simulink model "ScriptDemo"  (R2022b)
settings: configuration reference "TmVcThermal_Configuration_sub" (kept outside this file)
undefined symbols (not defined in the file): aaaa, bbbb, cTmComprCtrl_D_u8HvacFlowTable_db, cTmComprCtrl_D_u8HvacFlowTable_sw, cTmComprCtrl_n_i16ChillCmpIMax, cTmComprCtrl_n_i16ChillCmpIMin, cTmComprCtrl_n_i16ChillCmpIMin666, cTmComprCtrl_n_i16ChillCmpPMax, cTmComprCtrl_n_i16ChillCmpPMin, cTmComprCtrl_n_i16CmpChillCoolRpmKiMax, cTmComprCtrl_n_i16CmpChillCoolRpmKiMin, cTmComprCtrl_n_i16CmpChillCoolRpmKpMax, cTmComprCtrl_n_i16CmpChillCoolRpmKpMin, cTmComprCtrl_n_i16CmpCoolRpmKiMax, cTmComprCtrl_n_i16CmpCoolRpmKiMin, cTmComprCtrl_n_i16CmpCoolRpmKpMax, cTmComprCtrl_n_i16CmpCoolRpmKpMin, cTmComprCtrl_n_i16SM4CmpHeatKiMax, cTmComprCtrl_n_i16SM4CmpHeatKiMin, cTmComprCtrl_n_i16SM4CmpHeatKpMax, cTmComprCtrl_n_i16SM4CmpHeatKpMin, cTmComprCtrl_n_i16SM5CmpHeatKiMax, cTmComprCtrl_n_i16SM5CmpHeatKiMin, cTmComprCtrl_n_i16SM5CmpHeatKpMax, cTmComprCtrl_n_i16SM5CmpHeatKpMin, cTmComprCtrl_n_i16SM6CmpHeatKiMax, cTmComprCtrl_n_i16SM6CmpHeatKiMin, cTmComprCtrl_n_i16SM6CmpHeatKpMax, cTmComprCtrl_n_i16SM6CmpHeatKpMin, cTmComprCtrl_n_u16CmpMaxSpdFanFltLimt, cTmComprCtrl_n_u16CmpMaxSpdLoSidePFltLimt, cTmComprCtrl_n_u16CmpMaxSpdSensorFltLimt, cTmComprCtrl_n_u16CompMinRpm, cTmComprCtrl_n_u16CompRpmIncThres, cTmComprCtrl_t_u16BattCooltFFPeriod, cTmComprCtrl_t_u16BattCooltPIPeriod, cTmComprCtrl_t_u16CmpCoolFFPeriod, cTmComprCtrl_t_u16CmpCoolPIPeriod, cTmComprCtrl_t_u16CoolCmpChillFFPeriod, cTmComprCtrl_t_u16CoolCmpChillPIPeriod, cTmComprCtrl_t_u16SM4CmpHeatFFPeriod, cTmComprCtrl_t_u16SM4CmpHeatPIPeriod, cTmComprCtrl_t_u16SM5CmpHeatFFPeriod, cTmComprCtrl_t_u16SM5CmpHeatPIPeriod, cTmComprCtrl_t_u16SM6CmpHeatFFPeriod, cTmComprCtrl_t_u16SM6CmpHeatPIPeriod, cTmComprCtrl_Te_EvapClearInteg, cTmComprCtrl_Te_i16HpReqTempSaturoffset, cTmComprCtrl_Te_i16SatLpReplaceDiff, cTmComprCtrl_Te_i16SM3BatDiffStartEvapDecOffset, cTmComprCtrl_Te_i16SM3EvapLo, cTmComprCtrl_Te_i16SM3TBatDiffEntEvapDecOffset, cTmComprCtrl_Te_i16SM3TBatDiffEntEvapDecOffsetQuit, cTmComprCtrl_Te_s32ErrCmpChillPIContinueCoolH, cTmComprCtrl_Te_s32ErrCmpChillPIContinueCoolL, cTmComprCtrl_Te_s32ErrCmpPIContinueChillH, cTmComprCtrl_Te_s32ErrCmpPIContinueChillL, cTmComprCtrl_Te_s32ErrCmpPIContinueCoolH, cTmComprCtrl_Te_s32ErrCmpPIContinueCoolL, cTmComprCtrl_Te_s32ErrCmpPIContinueHeatH ... (+398)
libraries: simulink x782, PCMULib x640, simulink_need_slupdate x4
(part 20 of 41)

== system ScriptDemo/Create/createMerge/After/SM1SM21/ID26245_SM1FF ==
  sTmIn_Te_s32HvBattCooltTReq : Inport
  sTmIn_D_u8DCChrgSt : Inport  Port=2  OutDataTypeStr=uint8
  sTmSigProces_D_u8HvBattCoolgReq : Inport  Port=3  OutDataTypeStr=uint8
  sTmSigProces_Te_s32TAmb : Inport  Port=4  OutDataTypeStr=single
  sTmIn_D_u8HeatPump : Inport  Port=5  OutDataTypeStr=uint8
  Enable : EnablePort
  1-D Lookup Table : Lookup_n-D  NumberOfTableDimensions=1  BreakpointsForDimension1=tTmComprCtrl_fac_s32SM1FFTFactor_X  BreakpointsForDimension1DataTypeStr=Inherit: Inherit from 'Breakpoint data'  Table=tTmComprCtrl_fac_s32SM1FFTFactor  TableDataTypeStr=Inherit: Inherit from 'Table data'  ExtrapMethod=Clip  InternalRulePriority=Speed  OutDataTypeStr=Inherit: Inherit via back propagation  RndMeth=Simplest  InputSameDT=off
  2-D Lookup Table : Lookup_n-D  BreakpointsForDimension1=mTmComprCtrl_n_u16FFBattCooltRpmNorm_Y  BreakpointsForDimension2=mTmComprCtrl_n_u16FFBattCooltRpmNorm_X  BreakpointsForDimension1DataTypeStr=Inherit: Inherit from 'Breakpoint data'  BreakpointsForDimension2DataTypeStr=Inherit: Inherit from 'Breakpoint data'  Table=mTmComprCtrl_n_u16FFBattCooltRpmNorm  TableDataTypeStr=Inherit: Inherit from 'Table data'  ExtrapMethod=Clip  InternalRulePriority=Speed  OutDataTypeStr=Inherit: Inherit via back propagation  RndMeth=Simplest  InputSameDT=off
      settings: InputPortMap=u0,u1
  2-D Lookup Table1 : Lookup_n-D  BreakpointsForDimension1=mTmComprCtrl_n_u16FFBattCooltRpmNormNhp_Y  BreakpointsForDimension2=mTmComprCtrl_n_u16FFBattCooltRpmNormNhp_X  BreakpointsForDimension1DataTypeStr=Inherit: Inherit from 'Breakpoint data'  BreakpointsForDimension2DataTypeStr=Inherit: Inherit from 'Breakpoint data'  Table=mTmComprCtrl_n_u16FFBattCooltRpmNormNhp  TableDataTypeStr=Inherit: Inherit from 'Table data'  ExtrapMethod=Clip  InternalRulePriority=Speed  OutDataTypeStr=Inherit: Inherit via back propagation  RndMeth=Simplest  InputSameDT=off
      settings: InputPortMap=u0,u1
  2-D Lookup Table2 : Lookup_n-D  LookupTableObject=mTmComprCtrl_n_u16FFBattCooltRpmCharging  BreakpointsForDimension1=mTmComprCtrl_n_u16FFBattCooltRpmChargingNhp_Y  BreakpointsForDimension2=mTmComprCtrl_n_u16FFBattCooltRpmChargingNhp_X  BreakpointsForDimension1DataTypeStr=Inherit: Inherit from 'Breakpoint data'  BreakpointsForDimension2DataTypeStr=Inherit: Inherit from 'Breakpoint data'  Table=mTmComprCtrl_n_u16FFBattCooltRpmChargingNhp  TableDataTypeStr=Inherit: Inherit from 'Table data'  ExtrapMethod=Clip  InternalRulePriority=Speed  OutDataTypeStr=Inherit: Inherit via back propagation  RndMeth=Simplest  InputSameDT=off
      settings: InputPortMap=u0,u1
  2-D Lookup Table3 : Lookup_n-D  LookupTableObject=mTmComprCtrl_n_u16FFBattCooltRpmCharging  BreakpointsForDimension1=mTmComprCtrl_n_u16FFBattCooltRpmCharging_Y  BreakpointsForDimension2=mTmComprCtrl_n_u16FFBattCooltRpmCharging_X  BreakpointsForDimension1DataTypeStr=Inherit: Inherit from 'Breakpoint data'  BreakpointsForDimension2DataTypeStr=Inherit: Inherit from 'Breakpoint data'  Table=mTmComprCtrl_n_u16FFBattCooltRpmCharging  TableDataTypeStr=Inherit: Inherit from 'Table data'  ExtrapMethod=Clip  InternalRulePriority=Speed  OutDataTypeStr=Inherit: Inherit via back propagation  RndMeth=Simplest  InputSameDT=off
      settings: InputPortMap=u0,u1
  2-D Lookup Table4 : Lookup_n-D  LookupTableObject=mTmComprCtrl_n_u16FFBattCooltRpmCharging  BreakpointsForDimension1=mTmComprCtrl_n_u16FFBattCooltRpmSuperCharging_Y  BreakpointsForDimension2=mTmComprCtrl_n_u16FFBattCooltRpmSuperCharging_X  BreakpointsForDimension1DataTypeStr=Inherit: Inherit from 'Breakpoint data'  BreakpointsForDimension2DataTypeStr=Inherit: Inherit from 'Breakpoint data'  Table=mTmComprCtrl_n_u16FFBattCooltRpmSuperCharging  TableDataTypeStr=Inherit: Inherit from 'Table data'  ExtrapMethod=Clip  InternalRulePriority=Speed  OutDataTypeStr=Inherit: Inherit via back propagation  RndMeth=Simplest  InputSameDT=off
      settings: InputPortMap=u0,u1
  2-D Lookup Table5 : Lookup_n-D  LookupTableObject=mTmComprCtrl_n_u16FFBattCooltRpmCharging  BreakpointsForDimension1=mTmComprCtrl_n_u16FFBattCooltRpmSuperChargingNhp_Y  BreakpointsForDimension2=mTmComprCtrl_n_u16FFBattCooltRpmSuperChargingNhp_X  BreakpointsForDimension1DataTypeStr=Inherit: Inherit from 'Breakpoint data'  BreakpointsForDimension2DataTypeStr=Inherit: Inherit from 'Breakpoint data'  Table=mTmComprCtrl_n_u16FFBattCooltRpmSuperChargingNhp  TableDataTypeStr=Inherit: Inherit from 'Table data'  ExtrapMethod=Clip  InternalRulePriority=Speed  OutDataTypeStr=Inherit: Inherit via back propagation  RndMeth=Simplest  InputSameDT=off
      settings: InputPortMap=u0,u1
  Compare To Constant : simulink/Logic and Bit Operations/Compare To Constant  relop===  const=2  OutDataTypeStr=boolean
  Multiport Switch : MultiPortSwitch  DataPortOrder=Specify indices  DataPortIndices={2,12}  DataPortForDefault=Additional data port  DiagnosticForDefault=None  SaturateOnIntegerOverflow=off  InputSameDT=off
  Multiport Switch1 : MultiPortSwitch  DataPortOrder=Specify indices  DataPortIndices={2,12}  DataPortForDefault=Additional data port  DiagnosticForDefault=None  SaturateOnIntegerOverflow=off  InputSameDT=off
  Product : Product  OutDataTypeStr=uint16
  Switch : Switch  Criteria=u2 ~= 0  SaturateOnIntegerOverflow=off  InputSameDT=off
  SM1FF : Outport
  wires:
  2-D Lookup Table4/1 -> Multiport Switch/4
  2-D Lookup Table3/1 -> Multiport Switch/3
  [sTmIn_D_u8DCChrgSt] -> Multiport Switch/1
  2-D Lookup Table/1 -> Multiport Switch/2
  [sTmSigProces_D_u8HvBattCoolgReq] -> 2-D Lookup Table4/1, 2-D Lookup Table3/1, 2-D Lookup Table/1
  [sTmIn_Te_s32HvBattCooltTReq] -> 2-D Lookup Table3/2, 2-D Lookup Table4/2, 2-D Lookup Table/2
  sTmIn_Te_s32HvBattCooltTReq/1 -> [sTmIn_Te_s32HvBattCooltTReq]
  sTmIn_D_u8DCChrgSt/1 -> [sTmIn_D_u8DCChrgSt]
  sTmSigProces_D_u8HvBattCoolgReq/1 -> [sTmSigProces_D_u8HvBattCoolgReq]
  [sTmSigProces_Te_s32TAmb] -> 1-D Lookup Table/1
  Switch/1 -> Product/1  "rTmComprCtrl_fac_s32SM1FFRaw"
  1-D Lookup Table/1 -> Product/2  "rTmComprCtrl_fac_s32SM1FFTFactor"
  Product/1 -> SM1FF/1  "SM1FF"
  sTmSigProces_Te_s32TAmb/1 -> [sTmSigProces_Te_s32TAmb]
  2-D Lookup Table5/1 -> Multiport Switch1/4
  2-D Lookup Table1/1 -> Multiport Switch1/2
  [sTmIn_D_u8DCChrgSt] -> Multiport Switch1/1
  2-D Lookup Table2/1 -> Multiport Switch1/3
  [sTmSigProces_D_u8HvBattCoolgReq] -> 2-D Lookup Table5/1, 2-D Lookup Table2/1, 2-D Lookup Table1/1
  [sTmIn_Te_s32HvBattCooltTReq] -> 2-D Lookup Table5/2, 2-D Lookup Table2/2, 2-D Lookup Table1/2
  Compare To Constant/1 -> Switch/2
  [sTmIn_D_u8HeatPump] -> Compare To Constant/1
  Multiport Switch/1 -> Switch/1
  Multiport Switch1/1 -> Switch/3
  sTmIn_D_u8HeatPump/1 -> [sTmIn_D_u8HeatPump]

== system ScriptDemo/Create/createMerge/After/SM1SM21/ID26247_SM1Error ==
  sTmIn_Te_s32HvBattCooltTReq : Inport
  sTmSigProces_Te_s32HvBattCooltTFilter : Inport  Port=2
  "NegAndPosCheck " : Subsystem  AncestorBlock=CustomLib/TempNegAndPosCheck
  Saturation : Saturate  UpperLimit=40  LowerLimit=12
  Terminator : Terminator
  rTmComprCtrl_Te_s32TempError : Outport  OutDataTypeStr=single
  wires:
  sTmSigProces_Te_s32HvBattCooltTFilter/1 -> "NegAndPosCheck "/2(Acture)
  sTmIn_Te_s32HvBattCooltTReq/1 -> Saturation/1
  "NegAndPosCheck "/2(Dvt_PosFlag) -> Terminator/1
  Saturation/1 -> "NegAndPosCheck "/1(SetPoint)
  "NegAndPosCheck "/1(Dvt) -> rTmComprCtrl_Te_s32TempError/1

== system ScriptDemo/Create/createMerge/After/SM1SM21/SM1FFEnable ==
  xTmComprCtrl_B_CompOnReqCompOn : Inport  OutDataTypeStr=boolean
  BevvFFPeriod : Subsystem  mask{CounterLim=cTmComprCtrl_t_u16BattCooltFFPeriod}
      mask DialogControl ParameterGroupVar Prompt: 参数
  Compare To Constant2 : simulink/Logic and Bit Operations/Compare To Constant  relop===  const=0  OutDataTypeStr=boolean
  Compare To Constant3 : simulink/Logic and Bit Operations/Compare To Constant  relop===  const=1  OutDataTypeStr=boolean
  Logical Operator3 : Logic  AllPortsSameDT=off  OutDataTypeStr=boolean
  Unit Delay : UnitDelay  SampleTime=-1  HasFrameUpgradeWarning=on
  SM1FFEnable_B_SM1FFEnable : Outport  OutDataTypeStr=boolean
  wires:
  Unit Delay/1 -> Compare To Constant2/1
  [xTmComprCtrl_B_CompOnReqCompOn] -> Compare To Constant3/1, Unit Delay/1
  Compare To Constant2/1 -> Logical Operator3/1
  Logical Operator3/1 -> BevvFFPeriod/1(Counter_Reset)
  Compare To Constant3/1 -> Logical Operator3/2
  BevvFFPeriod/1(Counter_Trig) -> SM1FFEnable_B_SM1FFEnable/1
  xTmComprCtrl_B_CompOnReqCompOn/1 -> [xTmComprCtrl_B_CompOnReqCompOn]

== system ScriptDemo/Create/createMerge/After/SM1SM21/SM1_Ki ==
  sTmSigProces_D_u8BattThermReq : Inport
  sTmIn_D_u8DCChrgSt : Inport  Port=2
  sTmSigProces_D_u8HvBattCoolgReq : Inport  Port=3
  rTmComprCtrl_Te_s32TempError : Inport  Port=4
  2-D Lookup Table10 : Lookup_n-D  LookupTableObject=mTmComprCtrl_n_u16FFBattCooltRpmCharging  BreakpointsForDimension1=mTmComprCtrl_n_u16KiBattCooltRpmSuperCharging_Y  BreakpointsForDimension2=mTmComprCtrl_n_u16KiBattCooltRpmSuperCharging_X  BreakpointsForDimension1DataTypeStr=Inherit: Inherit from 'Breakpoint data'  BreakpointsForDimension2DataTypeStr=Inherit: Inherit from 'Breakpoint data'  Table=mTmComprCtrl_n_u16KiBattCooltRpmSuperCharging  TableDataTypeStr=Inherit: Inherit from 'Table data'  ExtrapMethod=Clip  InternalRulePriority=Speed  OutDataTypeStr=Inherit: Inherit via back propagation  RndMeth=Simplest  InputSameDT=off
      settings: InputPortMap=u0,u1
  2-D Lookup Table8 : Lookup_n-D  LookupTableObject=mTmComprCtrl_n_u16FFBattCooltRpmCharging  BreakpointsForDimension1=mTmComprCtrl_n_u16KiBattCooltRpmNorm_Y  BreakpointsForDimension2=mTmComprCtrl_n_u16KiBattCooltRpmNorm_X  BreakpointsForDimension1DataTypeStr=Inherit: Inherit from 'Breakpoint data'  BreakpointsForDimension2DataTypeStr=Inherit: Inherit from 'Breakpoint data'  Table=mTmComprCtrl_n_u16KiBattCooltRpmNorm  TableDataTypeStr=Inherit: Inherit from 'Table data'  ExtrapMethod=Clip  InternalRulePriority=Speed  OutDataTypeStr=Inherit: Inherit via back propagation  RndMeth=Simplest  InputSameDT=off
      settings: InputPortMap=u0,u1
  2-D Lookup Table9 : Lookup_n-D  LookupTableObject=mTmComprCtrl_n_u16FFBattCooltRpmCharging  BreakpointsForDimension1=mTmComprCtrl_n_u16KiBattCooltRpmCharging_Y  BreakpointsForDimension2=mTmComprCtrl_n_u16KiBattCooltRpmCharging_X  BreakpointsForDimension1DataTypeStr=Inherit: Inherit from 'Breakpoint data'  BreakpointsForDimension2DataTypeStr=Inherit: Inherit from 'Breakpoint data'  Table=mTmComprCtrl_n_u16KiBattCooltRpmCharging  TableDataTypeStr=Inherit: Inherit from 'Table data'  ExtrapMethod=Clip  InternalRulePriority=Speed  OutDataTypeStr=Inherit: Inherit via back propagation  RndMeth=Simplest  InputSameDT=off
      settings: InputPortMap=u0,u1
  tableChoose : Subsystem
  SM1Ki : Outport
  wires:
  sTmIn_D_u8DCChrgSt/1 -> tableChoose/2(sTmIn_D_u8DCChrgSt)
  sTmSigProces_D_u8BattThermReq/1 -> tableChoose/1(sTmSigProces_D_u8BattThermReq)
  2-D Lookup Table10/1 -> tableChoose/5(tab3)
  2-D Lookup Table8/1 -> tableChoose/3(tab1)
  2-D Lookup Table9/1 -> tableChoose/4(tab2)
  sTmSigProces_D_u8HvBattCoolgReq/1 -> 2-D Lookup Table8/1, 2-D Lookup Table10/1, 2-D Lookup Table9/1
  rTmComprCtrl_Te_s32TempError/1 -> 2-D Lookup Table8/2, 2-D Lookup Table10/2, 2-D Lookup Table9/2
  tableChoose/1(out) -> SM1Ki/1

== system ScriptDemo/Create/createMerge/After/SM1SM21/SM1_Kp ==
  sTmSigProces_D_u8BattThermReq : Inport
  sTmIn_D_u8DCChrgSt : Inport  Port=2
  sTmSigProces_D_u8HvBattCoolgReq : Inport  Port=3
  rTmComprCtrl_Te_s32TempError : Inport  Port=4
  2-D Lookup Table5 : Lookup_n-D  LookupTableObject=mTmComprCtrl_n_u16FFBattCooltRpmCharging  BreakpointsForDimension1=mTmComprCtrl_n_u16KpBattCooltRpmNorm_Y  BreakpointsForDimension2=mTmComprCtrl_n_u16KpBattCooltRpmNorm_X  BreakpointsForDimension1DataTypeStr=Inherit: Inherit from 'Breakpoint data'  BreakpointsForDimension2DataTypeStr=Inherit: Inherit from 'Breakpoint data'  Table=mTmComprCtrl_n_u16KpBattCooltRpmNorm  TableDataTypeStr=Inherit: Inherit from 'Table data'  ExtrapMethod=Clip  InternalRulePriority=Speed  OutDataTypeStr=Inherit: Inherit via back propagation  RndMeth=Simplest  InputSameDT=off
      settings: InputPortMap=u0,u1
  2-D Lookup Table6 : Lookup_n-D  LookupTableObject=mTmComprCtrl_n_u16FFBattCooltRpmCharging  BreakpointsForDimension1=mTmComprCtrl_n_u16KpBattCooltRpmCharging_Y  BreakpointsForDimension2=mTmComprCtrl_n_u16KpBattCooltRpmCharging_X  BreakpointsForDimension1DataTypeStr=Inherit: Inherit from 'Breakpoint data'  BreakpointsForDimension2DataTypeStr=Inherit: Inherit from 'Breakpoint data'  Table=mTmComprCtrl_n_u16KpBattCooltRpmCharging  TableDataTypeStr=Inherit: Inherit from 'Table data'  ExtrapMethod=Clip  InternalRulePriority=Speed  OutDataTypeStr=Inherit: Inherit via back propagation  RndMeth=Simplest  InputSameDT=off
      settings: InputPortMap=u0,u1
  2-D Lookup Table7 : Lookup_n-D  LookupTableObject=mTmComprCtrl_n_u16FFBattCooltRpmCharging  BreakpointsForDimension1=mTmComprCtrl_n_u16KpBattCooltRpmSuperCharging_Y  BreakpointsForDimension2=mTmComprCtrl_n_u16KpBattCooltRpmSuperCharging_X  BreakpointsForDimension1DataTypeStr=Inherit: Inherit from 'Breakpoint data'  BreakpointsForDimension2DataTypeStr=Inherit: Inherit from 'Breakpoint data'  Table=mTmComprCtrl_n_u16KpBattCooltRpmSuperCharging  TableDataTypeStr=Inherit: Inherit from 'Table data'  ExtrapMethod=Clip  InternalRulePriority=Speed  OutDataTypeStr=Inherit: Inherit via back propagation  RndMeth=Simplest  InputSameDT=off
      settings: InputPortMap=u0,u1
  tableChoose : Subsystem
  SM1Kp : Outport
  wires:
  sTmIn_D_u8DCChrgSt/1 -> tableChoose/2(sTmIn_D_u8DCChrgSt)
  sTmSigProces_D_u8BattThermReq/1 -> tableChoose/1(sTmSigProces_D_u8BattThermReq)
  2-D Lookup Table7/1 -> tableChoose/5(tab3)
  2-D Lookup Table5/1 -> tableChoose/3(tab1)
  2-D Lookup Table6/1 -> tableChoose/4(tab2)
  sTmSigProces_D_u8HvBattCoolgReq/1 -> 2-D Lookup Table7/1, 2-D Lookup Table6/1, 2-D Lookup Table5/1
  rTmComprCtrl_Te_s32TempError/1 -> 2-D Lookup Table7/2, 2-D Lookup Table6/2, 2-D Lookup Table5/2
  tableChoose/1(out) -> SM1Kp/1

== system ScriptDemo/Create/createMerge/After/SM2SM22/ID26239_SM2Error ==
  note: 控制对象为低压饱和温度
  note: 控制对象为蒸发器温度滤波值
  sTmSigProces_Te_s32EvapFanReqRamp : Inport  OutDataTypeStr=single
  sTmDiag_D_u8TeEvapFltSt : Inport  Port=2  OutDataTypeStr=uint8
  sTmSigProces_Te_s32EvapFanFilter : Inport  Port=3  OutDataTypeStr=single
  sTmSigProces_Te_s32SatLp : Inport  Port=4  OutDataTypeStr=single
  yTmRefriModeMgr_B_CoolOCRMode : Inport  Port=5  OutDataTypeStr=boolean
  Add : Sum  Inputs=+-  OutDataTypeStr=single
  Compare To Constant : simulink/Logic and Bit Operations/Compare To Constant  relop===  const=1  OutDataTypeStr=boolean
  Constant : Constant  Value=3  OutDataTypeStr=single
  Constant2 : Constant  Value=cTmComprCtrl_Te_i16SatLpReplaceDiff  OutDataTypeStr=int16
  NegAndPosCheck 1 : Subsystem  AncestorBlock=CustomLib/TempNegAndPosCheck
  Saturation1 : Saturate  UpperLimit=12  LowerLimit=3
  Switch1 : Switch  Criteria=u2 ~= 0  SaturateOnIntegerOverflow=off  InputSameDT=off
  Switch2 : Switch  Criteria=u2 ~= 0  SaturateOnIntegerOverflow=off  InputSameDT=off
  Terminator : Terminator
  rTmComprCtrl_Te_s32TempError : Outport
  wires:
  [sTmDiag_D_u8TeEvapFltSt] -> Switch1/2
  [sTmSigProces_Te_s32SatLp] -> Add/1
  Constant2/1 -> Add/2
  Switch2/1 -> Saturation1/1
  NegAndPosCheck 1/2(Dvt_PosFlag) -> Terminator/1
  NegAndPosCheck 1/1(Dvt) -> rTmComprCtrl_Te_s32TempError/1
  Add/1 -> Switch1/1
  Saturation1/1 -> NegAndPosCheck 1/1(SetPoint)  "rTmComprCtrl_Te_s32EvapTarget"
  sTmSigProces_Te_s32EvapFanReqRamp/1 -> [sTmSigProces_Te_s32EvapFanReqRamp]  "sTmSigProces_Te_s32EvapFanReqRamp"
  sTmDiag_D_u8TeEvapFltSt/1 -> [sTmDiag_D_u8TeEvapFltSt]  "sTmDiag_D_u8TeEvapFltSt"
  sTmSigProces_Te_s32EvapFanFilter/1 -> [sTmSigProces_Te_s32EvapFanFilter]  "sTmSigProces_Te_s32EvapFanFilter"
  sTmSigProces_Te_s32SatLp/1 -> [sTmSigProces_Te_s32SatLp]  "sTmSigProces_Te_s32SatLp"
  [yTmRefriModeMgr_B_CoolOCRMode] -> Compare To Constant/1
  Compare To Constant/1 -> Switch2/2
  Constant/1 -> Switch2/1
  yTmRefriModeMgr_B_CoolOCRMode/1 -> [yTmRefriModeMgr_B_CoolOCRMode]  "yTmRefriModeMgr_B_CoolOCRMode"
  [sTmSigProces_Te_s32EvapFanReqRamp] -> Switch2/3
  [sTmSigProces_Te_s32EvapFanFilter] -> Switch1/3
  Switch1/1 -> NegAndPosCheck 1/2(Acture)

== system ScriptDemo/Create/createMerge/After/SM2SM22/ID26267_SM2FF ==
  note: FF
  sTmSigProces_Te_s32EvapFanReqRamp : Inport  OutDataTypeStr=single
  sTmSigProces_Te_s32TAmb : Inport  Port=2  OutDataTypeStr=single
  sTmIn_X_s32ClimtRcirc : Inport  Port=3  OutDataTypeStr=single
  sTmComprCtrl_D_u8HvacFlowLevel : Inport  Port=4  OutDataTypeStr=uint8
  sTmIn_D_u8HeatPump : Inport  Port=5  OutDataTypeStr=uint8
  Enable : EnablePort
  Compare To Constant : simulink/Logic and Bit Operations/Compare To Constant  relop===  const=2  OutDataTypeStr=boolean
  Demux : Demux  Outputs=2
  Flow2RpmOsa : Subsystem  mask{BlwHeatLevel_db=cTmComprCtrl_D_u8HvacFlowTable_db, BlwHeatLevel_sw=cTmComprCtrl_D_u8HvacFlowTable_sw, FFBlw1=mTmComprCtrl_n_u16FFCmpCoolRpm_OsaFlow1, FFBlw1_Y=mTmComprCtrl_n_u16FFCmpCoolRpm_OsaFlow1_Y, FFBlw1_X=mTmComprCtrl_n_u16FFCmpCoolRpm_OsaFlow1_X, FFBlw3=mTmComprCtrl_n_u16FFCmpCoolRpm_OsaFlow3, FFBlw3_Y=mTmComprCtrl_n_u16FFCmpCoolRpm_OsaFlow3_Y, FFBlw3_X=mTmComprCtrl_n_u16FFCmpCoolRpm_OsaFlow3_X, FFBlw5=mTmComprCtrl_n_u16FFCmpCoolRpm_OsaFlow5, FFBlw5_Y=mTmComprCtrl_n_u16FFCmpCoolRpm_OsaFlow5_Y, FFBlw5_X=mTmComprCtrl_n_u16FFCmpCoolRpm_OsaFlow5_X, FFBlw7=mTmComprCtrl_n_u16FFCmpCoolRpm_OsaFlow7, FFBlw7_Y=mTmComprCtrl_n_u16FFCmpCoolRpm_OsaFlow7_Y, FFBlw7_X=mTmComprCtrl_n_u16FFCmpCoolRpm_OsaFlow7_X, FFBlw9=mTmComprCtrl_n_u16FFCmpCoolRpm_OsaFlow9, FFBlw9_Y=mTmComprCtrl_n_u16FFCmpCoolRpm_OsaFlow9_Y, FFBlw9_X=mTmComprCtrl_n_u16FFCmpCoolRpm_OsaFlow9_X}
      mask DialogControl ParameterGroupVar Prompt: 参数
  Flow2RpmOsa1 : Subsystem  mask{BlwHeatLevel_db=cTmComprCtrl_D_u8HvacFlowTable_db, BlwHeatLevel_sw=cTmComprCtrl_D_u8HvacFlowTable_sw, FFBlw1=mTmComprCtrl_n_u16FFCmpCoolRpmNhpOsaFlow1, FFBlw1_Y=mTmComprCtrl_n_u16FFCmpCoolRpmNhpOsaFlow1_Y, FFBlw1_X=mTmComprCtrl_n_u16FFCmpCoolRpmNhpOsaFlow1_X, FFBlw3=mTmComprCtrl_n_u16FFCmpCoolRpmNhpOsaFlow3, FFBlw3_Y=mTmComprCtrl_n_u16FFCmpCoolRpmNhpOsaFlow3_Y, FFBlw3_X=mTmComprCtrl_n_u16FFCmpCoolRpmNhpOsaFlow3_X, FFBlw5=mTmComprCtrl_n_u16FFCmpCoolRpmNhpOsaFlow5, FFBlw5_Y=mTmComprCtrl_n_u16FFCmpCoolRpmNhpOsaFlow5_Y, FFBlw5_X=mTmComprCtrl_n_u16FFCmpCoolRpmNhpOsaFlow5_X, FFBlw7=mTmComprCtrl_n_u16FFCmpCoolRpmNhpOsaFlow7, FFBlw7_Y=mTmComprCtrl_n_u16FFCmpCoolRpmNhpOsaFlow7_Y, FFBlw7_X=mTmComprCtrl_n_u16FFCmpCoolRpmNhpOsaFlow7_X, FFBlw9=mTmComprCtrl_n_u16FFCmpCoolRpmNhpOsaFlow9, FFBlw9_Y=mTmComprCtrl_n_u16FFCmpCoolRpmNhpOsaFlow9_Y, FFBlw9_X=mTmComprCtrl_n_u16FFCmpCoolRpmNhpOsaFlow9_X}
      mask DialogControl ParameterGroupVar Prompt: 参数
  Flow2RpmRec : Subsystem  mask{BlwHeatLevel_db=cTmComprCtrl_D_u8HvacFlowTable_db, BlwHeatLevel_sw=cTmComprCtrl_D_u8HvacFlowTable_sw, FFBlw1=mTmComprCtrl_n_u16FFCmpCoolRpm_RecFlow1, FFBlw1_Y=mTmComprCtrl_n_u16FFCmpCoolRpm_RecFlow1_Y, FFBlw1_X=mTmComprCtrl_n_u16FFCmpCoolRpm_RecFlow1_X, FFBlw3=mTmComprCtrl_n_u16FFCmpCoolRpm_RecFlow3, FFBlw3_Y=mTmComprCtrl_n_u16FFCmpCoolRpm_RecFlow3_Y, FFBlw3_X=mTmComprCtrl_n_u16FFCmpCoolRpm_RecFlow3_X, FFBlw5=mTmComprCtrl_n_u16FFCmpCoolRpm_RecFlow5, FFBlw5_Y=mTmComprCtrl_n_u16FFCmpCoolRpm_RecFlow5_Y, FFBlw5_X=mTmComprCtrl_n_u16FFCmpCoolRpm_RecFlow5_X, FFBlw7=mTmComprCtrl_n_u16FFCmpCoolRpm_RecFlow7, FFBlw7_Y=mTmComprCtrl_n_u16FFCmpCoolRpm_RecFlow7_Y, FFBlw7_X=mTmComprCtrl_n_u16FFCmpCoolRpm_RecFlow7_X, FFBlw9=mTmComprCtrl_n_u16FFCmpCoolRpm_RecFlow9, FFBlw9_Y=mTmComprCtrl_n_u16FFCmpCoolRpm_RecFlow9_Y, FFBlw9_X=mTmComprCtrl_n_u16FFCmpCoolRpm_RecFlow9_X}
      mask DialogControl ParameterGroupVar Prompt: 参数
  Flow2RpmRec1 : Subsystem  mask{BlwHeatLevel_db=cTmComprCtrl_D_u8HvacFlowTable_db, BlwHeatLevel_sw=cTmComprCtrl_D_u8HvacFlowTable_sw, FFBlw1=mTmComprCtrl_n_u16FFCmpCoolRpmNhpRecFlow1, FFBlw1_Y=mTmComprCtrl_n_u16FFCmpCoolRpmNhpRecFlow1_Y, FFBlw1_X=mTmComprCtrl_n_u16FFCmpCoolRpmNhpRecFlow1_X, FFBlw3=mTmComprCtrl_n_u16FFCmpCoolRpmNhpRecFlow3, FFBlw3_Y=mTmComprCtrl_n_u16FFCmpCoolRpmNhpRecFlow3_Y, FFBlw3_X=mTmComprCtrl_n_u16FFCmpCoolRpmNhpRecFlow3_X, FFBlw5=mTmComprCtrl_n_u16FFCmpCoolRpmNhpRecFlow5, FFBlw5_Y=mTmComprCtrl_n_u16FFCmpCoolRpmNhpRecFlow5_Y, FFBlw5_X=mTmComprCtrl_n_u16FFCmpCoolRpmNhpRecFlow5_X, FFBlw7=mTmComprCtrl_n_u16FFCmpCoolRpmNhpRecFlow7, FFBlw7_Y=mTmComprCtrl_n_u16FFCmpCoolRpmNhpRecFlow7_Y, FFBlw7_X=mTmComprCtrl_n_u16FFCmpCoolRpmNhpRecFlow7_X, FFBlw9=mTmComprCtrl_n_u16FFCmpCoolRpmNhpRecFlow9, FFBlw9_Y=mTmComprCtrl_n_u16FFCmpCoolRpmNhpRecFlow9_Y, FFBlw9_X=mTmComprCtrl_n_u16FFCmpCoolRpmNhpRecFlow9_X}
      mask DialogControl ParameterGroupVar Prompt: 参数
  Mux : Mux  Inputs=2
  Mux1 : Mux  Inputs=2
  Signal Conversion : SignalConversion  OverrideOpt=off
  Signal Conversion1 : SignalConversion  OverrideOpt=off
  Switch : Switch  Criteria=u2 ~= 0  SaturateOnIntegerOverflow=off  InputSameDT=off
  interpolation : PCMULib/Calculation/interpolation  SystemSampleTime=-1  VariantActivationTime=update diagram  Latency=0  AutoFrameSizeCalculation=off
      settings: SourceProductName=PCMULib
  SM2FF : Outport  OutDataTypeStr=uint16
  wires:
  [sTmIn_X_s32ClimtRcirc] -> interpolation/1
  interpolation/1 -> SM2FF/1
  sTmSigProces_Te_s32EvapFanReqRamp/1 -> [sTmSigProces_Te_s32EvapFanReqRamp]
  sTmSigProces_Te_s32TAmb/1 -> [sTmSigProces_Te_s32TAmb]
  sTmIn_X_s32ClimtRcirc/1 -> [sTmIn_X_s32ClimtRcirc]
  sTmComprCtrl_D_u8HvacFlowLevel/1 -> [sTmComprCtrl_D_u8HvacFlowLevel]
  [sTmComprCtrl_D_u8HvacFlowLevel] -> Flow2RpmRec/1(md_u8Blw)
  [sTmSigProces_Te_s32TAmb] -> Flow2RpmRec/2(breakpoint1)
  [sTmSigProces_Te_s32EvapFanReqRamp] -> Flow2RpmRec/3(breakpoint2)
  [sTmComprCtrl_D_u8HvacFlowLevel] -> Flow2RpmOsa/1(md_u8Blw)
  [sTmSigProces_Te_s32EvapFanReqRamp] -> Flow2RpmOsa/3(breakpoint2)
  [sTmSigProces_Te_s32TAmb] -> Flow2RpmOsa/2(breakpoint1)
  [sTmIn_D_u8HeatPump] -> Compare To Constant/1
  Compare To Constant/1 -> Switch/2
  Flow2RpmOsa/1(Flow2Rpm) -> Mux/2
  Flow2RpmRec/1(Flow2Rpm) -> Mux/1
  Mux/1 -> Switch/1
  [sTmSigProces_Te_s32TAmb] -> Flow2RpmOsa1/2(breakpoint1)
  [sTmSigProces_Te_s32TAmb] -> Flow2RpmRec1/2(breakpoint1)
  [sTmSigProces_Te_s32EvapFanReqRamp] -> Flow2RpmRec1/3(breakpoint2)
  [sTmComprCtrl_D_u8HvacFlowLevel] -> Flow2RpmRec1/1(md_u8Blw)
  [sTmSigProces_Te_s32EvapFanReqRamp] -> Flow2RpmOsa1/3(breakpoint2)
  [sTmComprCtrl_D_u8HvacFlowLevel] -> Flow2RpmOsa1/1(md_u8Blw)
  Flow2RpmRec1/1(Flow2Rpm) -> Mux1/1
  Flow2RpmOsa1/1(Flow2Rpm) -> Mux1/2
  Mux1/1 -> Switch/3
  Demux/2 -> Signal Conversion1/1
  Demux/1 -> Signal Conversion/1
  sTmIn_D_u8HeatPump/1 -> [sTmIn_D_u8HeatPump]
  Signal Conversion/1 -> interpolation/2  "rTmComprCtrl_n_u16ComprRpmFFSM2Rec"
  Signal Conversion1/1 -> interpolation/3  "rTmComprCtrl_n_u16ComprRpmFFSM2Osa"
  Switch/1 -> Demux/1

== system ScriptDemo/Create/createMerge/After/SM2SM22/SM2FFEnable ==
  xTmComprCtrl_B_CompOnReqCompOn : Inport  OutDataTypeStr=boolean
  Compare To Constant2 : simulink/Logic and Bit Operations/Compare To Constant  relop===  const=0  OutDataTypeStr=boolean
  Compare To Constant3 : simulink/Logic and Bit Operations/Compare To Constant  relop===  const=1  OutDataTypeStr=boolean
  Logical Operator3 : Logic  AllPortsSameDT=off  OutDataTypeStr=boolean
  PeriodTrig : Subsystem  mask{CounterLim=cTmComprCtrl_t_u16CmpCoolFFPeriod}
      mask DialogControl ParameterGroupVar Prompt: 参数
  Unit Delay : UnitDelay  SampleTime=-1  HasFrameUpgradeWarning=on
  SM2FFEnable_B_SM2FFEnable : Outport  OutDataTypeStr=boolean
  wires:
  Unit Delay/1 -> Compare To Constant2/1
  [xTmComprCtrl_B_CompOnReqCompOn] -> Compare To Constant3/1, Unit Delay/1
  Compare To Constant2/1 -> Logical Operator3/1
  Logical Operator3/1 -> PeriodTrig/1(Counter_Reset)
  Compare To Constant3/1 -> Logical Operator3/2
  xTmComprCtrl_B_CompOnReqCompOn/1 -> [xTmComprCtrl_B_CompOnReqCompOn]
  PeriodTrig/1(Counter_Trig) -> SM2FFEnable_B_SM2FFEnable/1

== system ScriptDemo/Create/createMerge/After/SM2SM22/SM2_Ki ==
  rTmComprCtrl_Te_s32TempError : Inport
  sTmSigProces_Te_s32TAmb : Inport  Port=2  OutDataTypeStr=single
  sTmIn_X_s32ClimtRcirc : Inport  Port=3  OutDataTypeStr=single
  sTmComprCtrl_D_u8HvacFlowLevel : Inport  Port=4  OutDataTypeStr=uint8
  Flow2Rpm : Subsystem  mask{BlwHeatLevel_db=cTmComprCtrl_D_u8HvacFlowTable_db, BlwHeatLevel_sw=cTmComprCtrl_D_u8HvacFlowTable_sw, FFBlw1=mTmComprCtrl_n_u16KiCmpCoolRpm_RecFlow1, FFBlw1_Y=mTmComprCtrl_n_u16KiCmpCoolRpm_RecFlow1_Y, FFBlw1_X=mTmComprCtrl_n_u16KiCmpCoolRpm_RecFlow1_X, FFBlw3=mTmComprCtrl_n_u16KiCmpCoolRpm_RecFlow3, FFBlw3_Y=mTmComprCtrl_n_u16KiCmpCoolRpm_RecFlow3_Y, FFBlw3_X=mTmComprCtrl_n_u16KiCmpCoolRpm_RecFlow3_X, FFBlw5=mTmComprCtrl_n_u16KiCmpCoolRpm_RecFlow5, FFBlw5_Y=mTmComprCtrl_n_u16KiCmpCoolRpm_RecFlow5_Y, FFBlw5_X=mTmComprCtrl_n_u16KiCmpCoolRpm_RecFlow5_X, FFBlw7=mTmComprCtrl_n_u16KiCmpCoolRpm_RecFlow7, FFBlw7_Y=mTmComprCtrl_n_u16KiCmpCoolRpm_RecFlow7_Y, FFBlw7_X=mTmComprCtrl_n_u16KiCmpCoolRpm_RecFlow7_X, FFBlw9=mTmComprCtrl_n_u16KiCmpCoolRpm_RecFlow9, FFBlw9_Y=mTmComprCtrl_n_u16KiCmpCoolRpm_RecFlow9_Y, FFBlw9_X=mTmComprCtrl_n_u16KiCmpCoolRpm_RecFlow9_X}
      mask DialogControl ParameterGroupVar Prompt: 参数
  Flow2Rpm1 : Subsystem  mask{BlwHeatLevel_db=cTmComprCtrl_D_u8HvacFlowTable_db, BlwHeatLevel_sw=cTmComprCtrl_D_u8HvacFlowTable_sw, FFBlw1=mTmComprCtrl_n_u16KiCmpCoolRpm_OsaFlow1, FFBlw1_Y=mTmComprCtrl_n_u16KiCmpCoolRpm_OsaFlow1_Y, FFBlw1_X=mTmComprCtrl_n_u16KiCmpCoolRpm_OsaFlow1_X, FFBlw3=mTmComprCtrl_n_u16KiCmpCoolRpm_OsaFlow3, FFBlw3_Y=mTmComprCtrl_n_u16KiCmpCoolRpm_OsaFlow3_Y, FFBlw3_X=mTmComprCtrl_n_u16KiCmpCoolRpm_OsaFlow3_X, FFBlw5=mTmComprCtrl_n_u16KiCmpCoolRpm_OsaFlow5, FFBlw5_Y=mTmComprCtrl_n_u16KiCmpCoolRpm_OsaFlow5_Y, FFBlw5_X=mTmComprCtrl_n_u16KiCmpCoolRpm_OsaFlow5_X, FFBlw7=mTmComprCtrl_n_u16KiCmpCoolRpm_OsaFlow7, FFBlw7_Y=mTmComprCtrl_n_u16KiCmpCoolRpm_OsaFlow7_Y, FFBlw7_X=mTmComprCtrl_n_u16KiCmpCoolRpm_OsaFlow7_X, FFBlw9=mTmComprCtrl_n_u16KiCmpCoolRpm_OsaFlow9, FFBlw9_Y=mTmComprCtrl_n_u16KiCmpCoolRpm_OsaFlow9_Y, FFBlw9_X=mTmComprCtrl_n_u16KiCmpCoolRpm_OsaFlow9_X}
      mask DialogControl ParameterGroupVar Prompt: 参数
  interpolation : PCMULib/Calculation/interpolation  SystemSampleTime=-1  VariantActivationTime=update diagram  Latency=0  AutoFrameSizeCalculation=off
      settings: SourceProductName=PCMULib
  SM2Ki : Outport
  wires:
  interpolation/1 -> SM2Ki/1
  [sTmIn_X_s32ClimtRcirc] -> interpolation/1
  rTmComprCtrl_Te_s32TempError/1 -> [rTmComprCtrl_Te_s32TempError]
  sTmSigProces_Te_s32TAmb/1 -> [sTmSigProces_Te_s32TAmb]
  sTmIn_X_s32ClimtRcirc/1 -> [sTmIn_X_s32ClimtRcirc]
  sTmComprCtrl_D_u8HvacFlowLevel/1 -> [sTmComprCtrl_D_u8HvacFlowLevel]
  [sTmComprCtrl_D_u8HvacFlowLevel] -> Flow2Rpm/1(md_u8Blw)
  [sTmSigProces_Te_s32TAmb] -> Flow2Rpm/2(breakpoint1)
  [rTmComprCtrl_Te_s32TempError] -> Flow2Rpm/3(breakpoint2)
  [sTmComprCtrl_D_u8HvacFlowLevel] -> Flow2Rpm1/1(md_u8Blw)
  [sTmSigProces_Te_s32TAmb] -> Flow2Rpm1/2(breakpoint1)
  [rTmComprCtrl_Te_s32TempError] -> Flow2Rpm1/3(breakpoint2)
  Flow2Rpm/1(Flow2Rpm) -> interpolation/2  "rTmComprCtrl_n_u16ComprRpmKiSM2Rec"
  Flow2Rpm1/1(Flow2Rpm) -> interpolation/3  "rTmComprCtrl_n_u16ComprRpmKiSM2Osa"

== system ScriptDemo/Create/createMerge/After/SM2SM22/SM2_Kp ==
  rTmComprCtrl_Te_s32TempError : Inport
  sTmSigProces_Te_s32TAmb : Inport  Port=2  OutDataTypeStr=single
  sTmIn_X_s32ClimtRcirc : Inport  Port=3  OutDataTypeStr=single
  sTmComprCtrl_D_u8HvacFlowLevel : Inport  Port=4  OutDataTypeStr=uint8
  Osa : Subsystem  mask{BlwHeatLevel_db=cTmComprCtrl_D_u8HvacFlowTable_db, BlwHeatLevel_sw=cTmComprCtrl_D_u8HvacFlowTable_sw, FFBlw1=mTmComprCtrl_n_u16KpCmpCoolRpm_OsaFlow1, FFBlw1_Y=mTmComprCtrl_n_u16KpCmpCoolRpm_OsaFlow1_Y, FFBlw1_X=mTmComprCtrl_n_u16KpCmpCoolRpm_OsaFlow1_X, FFBlw3=mTmComprCtrl_n_u16KpCmpCoolRpm_OsaFlow3, FFBlw3_Y=mTmComprCtrl_n_u16KpCmpCoolRpm_OsaFlow3_Y, FFBlw3_X=mTmComprCtrl_n_u16KpCmpCoolRpm_OsaFlow3_X, FFBlw5=mTmComprCtrl_n_u16KpCmpCoolRpm_OsaFlow5, FFBlw5_Y=mTmComprCtrl_n_u16KpCmpCoolRpm_OsaFlow5_Y, FFBlw5_X=mTmComprCtrl_n_u16KpCmpCoolRpm_OsaFlow5_X, FFBlw7=mTmComprCtrl_n_u16KpCmpCoolRpm_OsaFlow7, FFBlw7_Y=mTmComprCtrl_n_u16KpCmpCoolRpm_OsaFlow7_Y, FFBlw7_X=mTmComprCtrl_n_u16KpCmpCoolRpm_OsaFlow7_X, FFBlw9=mTmComprCtrl_n_u16KpCmpCoolRpm_OsaFlow9, FFBlw9_Y=mTmComprCtrl_n_u16KpCmpCoolRpm_OsaFlow9_Y, FFBlw9_X=mTmComprCtrl_n_u16KpCmpCoolRpm_OsaFlow9_X}
      mask DialogControl ParameterGroupVar Prompt: 参数
  Rec : Subsystem  mask{BlwHeatLevel_db=cTmComprCtrl_D_u8HvacFlowTable_db, BlwHeatLevel_sw=cTmComprCtrl_D_u8HvacFlowTable_sw, FFBlw1=mTmComprCtrl_n_u16KpCmpCoolRpm_RecFlow1, FFBlw1_Y=mTmComprCtrl_n_u16KpCmpCoolRpm_RecFlow1_Y, FFBlw1_X=mTmComprCtrl_n_u16KpCmpCoolRpm_RecFlow1_X, FFBlw3=mTmComprCtrl_n_u16KpCmpCoolRpm_RecFlow3, FFBlw3_Y=mTmComprCtrl_n_u16KpCmpCoolRpm_RecFlow3_Y, FFBlw3_X=mTmComprCtrl_n_u16KpCmpCoolRpm_RecFlow3_X, FFBlw5=mTmComprCtrl_n_u16KpCmpCoolRpm_RecFlow5, FFBlw5_Y=mTmComprCtrl_n_u16KpCmpCoolRpm_RecFlow5_Y, FFBlw5_X=mTmComprCtrl_n_u16KpCmpCoolRpm_RecFlow5_X, FFBlw7=mTmComprCtrl_n_u16KpCmpCoolRpm_RecFlow7, FFBlw7_Y=mTmComprCtrl_n_u16KpCmpCoolRpm_RecFlow7_Y, FFBlw7_X=mTmComprCtrl_n_u16KpCmpCoolRpm_RecFlow7_X, FFBlw9=mTmComprCtrl_n_u16KpCmpCoolRpm_RecFlow9, FFBlw9_Y=mTmComprCtrl_n_u16KpCmpCoolRpm_RecFlow9_Y, FFBlw9_X=mTmComprCtrl_n_u16KpCmpCoolRpm_RecFlow9_X}
      mask DialogControl ParameterGroupVar Prompt: 参数
  interpolation : PCMULib/Calculation/interpolation  SystemSampleTime=-1  VariantActivationTime=update diagram  Latency=0  AutoFrameSizeCalculation=off
      settings: SourceProductName=PCMULib
  SM2Kp : Outport
  wires:
  interpolation/1 -> SM2Kp/1
  [sTmIn_X_s32ClimtRcirc] -> interpolation/1
  rTmComprCtrl_Te_s32TempError/1 -> [rTmComprCtrl_Te_s32TempError]
  sTmSigProces_Te_s32TAmb/1 -> [sTmSigProces_Te_s32TAmb]
  sTmIn_X_s32ClimtRcirc/1 -> [sTmIn_X_s32ClimtRcirc]
  sTmComprCtrl_D_u8HvacFlowLevel/1 -> [sTmComprCtrl_D_u8HvacFlowLevel]
  [sTmComprCtrl_D_u8HvacFlowLevel] -> Rec/1(md_u8Blw)
  [sTmSigProces_Te_s32TAmb] -> Rec/2(breakpoint1)
  [rTmComprCtrl_Te_s32TempError] -> Rec/3(breakpoint2)
  [sTmComprCtrl_D_u8HvacFlowLevel] -> Osa/1(md_u8Blw)
  [sTmSigProces_Te_s32TAmb] -> Osa/2(breakpoint1)
  [rTmComprCtrl_Te_s32TempError] -> Osa/3(breakpoint2)
  Rec/1(Flow2Rpm) -> interpolation/2  "rTmComprCtrl_n_u16ComprRpmKpSM2Rec"
  Osa/1(Flow2Rpm) -> interpolation/3  "rTmComprCtrl_n_u16ComprRpmKpSM2Osa"

== system ScriptDemo/Create/createMerge/After/SM3SM23/ID26262_SM3FF ==
  note: 0704：这里为什么用误差来查表？
  sTmIn_Te_s32HvBattCooltTReq : Inport
  sTmSigProces_Te_s32EvapFanReqRamp : Inport  Port=2  OutDataTypeStr=single
  sTmIn_D_u8DCChrgSt : Inport  Port=3  OutDataTypeStr=uint8
  sTmSigProces_Te_s32TAmb : Inport  Port=4  OutDataTypeStr=single
  sTmIn_Te_s32BattHv : Inport  Port=5  OutDataTypeStr=single
  sTmIn_X_s32ClimtRcirc : Inport  Port=6  OutDataTypeStr=single
  sTmComprCtrl_D_u8HvacFlowLevel : Inport  Port=7  OutDataTypeStr=uint8
  sTmSigProces_D_u8HvBattCoolgReq : Inport  Port=8  OutDataTypeStr=uint8
  xTmComprCtrl_B_CompOnReqCompOn : Inport  Port=9  OutDataTypeStr=boolean
  sTmIn_D_u8HeatPump : Inport  Port=10  OutDataTypeStr=uint8
  1-D Lookup Table1 : Lookup_n-D  NumberOfTableDimensions=1  BreakpointsForDimension1=tTmComprCtrl_n_s32Kcmp_X  BreakpointsForDimension1DataTypeStr=Inherit: Inherit from 'Breakpoint data'  Table=tTmComprCtrl_n_s32Kcmp  TableDataTypeStr=Inherit: Inherit from 'Table data'  ExtrapMethod=Clip  InternalRulePriority=Speed  OutDataTypeStr=Inherit: Inherit via back propagation  RndMeth=Simplest  InputSameDT=off
  1-D Lookup Table2 : Lookup_n-D  NumberOfTableDimensions=1  BreakpointsForDimension1=tTmComprCtrl_n_s32KChill_X  BreakpointsForDimension1DataTypeStr=Inherit: Inherit from 'Breakpoint data'  Table=tTmComprCtrl_n_s32KChill  TableDataTypeStr=Inherit: Inherit from 'Table data'  ExtrapMethod=Clip  InternalRulePriority=Speed  OutDataTypeStr=Inherit: Inherit via back propagation  RndMeth=Simplest  InputSameDT=off
  Add : Sum  OutDataTypeStr=uint16
  From7 : From  Commented=on  GotoTag=sTmIn_Te_s32HvBattCooltTReq
  Product : Product
  Product1 : Product
  SM1FFEnable : Subsystem
  SM2FFEnable : Subsystem
  SM3SM1FF : Subsystem
  SM3SM2FF : Subsystem
  SM3FF : Outport
  wires:
  [sTmIn_Te_s32BattHv] -> 1-D Lookup Table2/1
  1-D Lookup Table1/1 -> Product1/1  "Kcmp"
  1-D Lookup Table2/1 -> Product/2  "KChill"
  [sTmSigProces_Te_s32TAmb] -> 1-D Lookup Table1/1
  Product/1 -> Add/1
  [SM1FF] -> Product/1
  Product1/1 -> Add/2
  [SM2FF] -> Product1/2
  Add/1 -> SM3FF/1
  sTmIn_Te_s32HvBattCooltTReq/1 -> [sTmIn_Te_s32HvBattCooltTReq]
  sTmSigProces_Te_s32EvapFanReqRamp/1 -> [sTmSigProces_Te_s32EvapFanReqRamp]
  sTmIn_D_u8DCChrgSt/1 -> [sTmIn_D_u8DCChrgSt]
  sTmSigProces_Te_s32TAmb/1 -> [sTmSigProces_Te_s32TAmb]
  sTmIn_Te_s32BattHv/1 -> [sTmIn_Te_s32BattHv]
  sTmIn_X_s32ClimtRcirc/1 -> [sTmIn_X_s32ClimtRcirc]
  sTmComprCtrl_D_u8HvacFlowLevel/1 -> [sTmComprCtrl_D_u8HvacFlowLevel]
  sTmSigProces_D_u8HvBattCoolgReq/1 -> [sTmSigProces_D_u8HvBattCoolgReq]
  SM1FFEnable/1(SM1FFEnable_B_SM1FFEnable) -> [SM1FFEnable_B_SM1FFEnable]
  [xTmComprCtrl_B_CompOnReqCompOn] -> SM1FFEnable/1(xTmComprCtrl_B_CompOnReqCompOn)
  [SM1FFEnable_B_SM1FFEnable] -> SM3SM1FF/Enable
  [sTmSigProces_D_u8HvBattCoolgReq] -> SM3SM1FF/3(sTmSigProces_D_u8HvBattCoolgReq)
  [sTmIn_D_u8DCChrgSt] -> SM3SM1FF/2(sTmIn_D_u8DCChrgSt)
  [sTmIn_Te_s32HvBattCooltTReq] -> SM3SM1FF/1(sTmIn_Te_s32HvBattCooltTReq)
  [SM2FFEnable_B_SM2FFEnable] -> SM3SM2FF/Enable
  [xTmComprCtrl_B_CompOnReqCompOn] -> SM2FFEnable/1(xTmComprCtrl_B_CompOnReqCompOn)
  SM2FFEnable/1(SM2FFEnable_B_SM2FFEnable) -> [SM2FFEnable_B_SM2FFEnable]
  SM3SM1FF/1(SM1FF) -> [SM1FF]  "rTmComprCtrl_n_u16ComprRpmFFSM3SM1"
  xTmComprCtrl_B_CompOnReqCompOn/1 -> [xTmComprCtrl_B_CompOnReqCompOn]
  [sTmSigProces_Te_s32TAmb] -> SM3SM1FF/4(sTmSigProces_Te_s32TAmb)
  SM3SM2FF/1(SM2FF) -> [SM2FF]  "rTmComprCtrl_n_u16ComprRpmFFSM3SM2"
  [sTmSigProces_Te_s32EvapFanReqRamp] -> SM3SM2FF/1(sTmSigProces_Te_s32EvapFanReqRamp)
  [sTmSigProces_Te_s32TAmb] -> SM3SM2FF/2(sTmSigProces_Te_s32TAmb)
  [sTmIn_X_s32ClimtRcirc] -> SM3SM2FF/3(sTmIn_X_s32ClimtRcirc)
  [sTmComprCtrl_D_u8HvacFlowLevel] -> SM3SM2FF/4(sTmComprCtrl_D_u8HvacFlowLevel)
  [sTmIn_D_u8HeatPump] -> SM3SM2FF/5(sTmIn_D_u8HeatPump)
  sTmIn_D_u8HeatPump/1 -> [sTmIn_D_u8HeatPump]
  [sTmIn_D_u8HeatPump] -> SM3SM1FF/5(sTmIn_D_u8HeatPump)

== system ScriptDemo/Create/createMerge/After/SM3SM23/ID26263_SM3Error ==
  note: 非热泵
  note: 1: 非热泵
      | 2：热泵
  note: 热泵
  sTmSigProces_Te_s32EvapFanReqRamp : Inport  OutDataTypeStr=single
  sTmIn_D_u8HeatPump : Inport  Port=2  OutDataTypeStr=uint8
  sTmIn_Te_s32HvBattCooltTReq : Inport  Port=3  OutDataTypeStr=single
  sTmSigProces_D_u8HvBattCoolgReq : Inport  Port=4  OutDataTypeStr=uint8
  sTmSigProces_Te_s32EvapFanFilter : Inport  Port=5  OutDataTypeStr=single
  sTmSigProces_Te_s32HvBattCooltTFilter : Inport  Port=6  OutDataTypeStr=single
  xTmComprCtrl_B_ModeChanged : Inport  Port=7  OutDataTypeStr=boolean
  Compare To Constant1 : simulink/Logic and Bit Operations/Compare To Constant  relop===  const=2  OutDataTypeStr=boolean
  SM3HPErr : Subsystem
  SM3NHPErr : Subsystem
  Switch : Switch  Criteria=u2 ~= 0  SaturateOnIntegerOverflow=off  InputSameDT=off
  rTmComprCtrl_Te_s32TempError : Outport
  wires:
  Compare To Constant1/1 -> Switch/2
  [sTmIn_D_u8HeatPump] -> Compare To Constant1/1
  Switch/1 -> rTmComprCtrl_Te_s32TempError/1
  SM3NHPErr/1(SM3NHPErr_Te_s32Error) -> Switch/3
  SM3HPErr/1(SM3HPErr_Te_s32Error) -> Switch/1
  [sTmSigProces_Te_s32EvapFanReqRamp] -> SM3HPErr/1(sTmSigProces_Te_s32EvapFanReqRamp)
  [sTmIn_Te_s32HvBattCooltTReq] -> SM3HPErr/2(sTmIn_Te_s32HvBattCooltTReq)
  [sTmSigProces_Te_s32EvapFanFilter] -> SM3HPErr/3(sTmSigProces_Te_s32EvapFanFilter)
  [sTmSigProces_Te_s32HvBattCooltTFilter] -> SM3HPErr/4(sTmSigProces_Te_s32HvBattCooltTFilter)
  [sTmSigProces_Te_s32EvapFanReqRamp] -> SM3NHPErr/1(sTmSigProces_Te_s32EvapFanReqRamp)
  [sTmIn_Te_s32HvBattCooltTReq] -> SM3NHPErr/2(sTmIn_Te_s32HvBattCooltTReq)
  [sTmSigProces_D_u8HvBattCoolgReq] -> SM3NHPErr/3(sTmSigProces_D_u8HvBattCoolgReq)
  [sTmSigProces_Te_s32EvapFanFilter] -> SM3NHPErr/4(sTmSigProces_Te_s32EvapFanFilter)
  [sTmSigProces_Te_s32HvBattCooltTFilter] -> SM3NHPErr/5(sTmSigProces_Te_s32HvBattCooltTFilter)
  sTmSigProces_Te_s32EvapFanReqRamp/1 -> [sTmSigProces_Te_s32EvapFanReqRamp]
  sTmIn_D_u8HeatPump/1 -> [sTmIn_D_u8HeatPump]
  sTmIn_Te_s32HvBattCooltTReq/1 -> [sTmIn_Te_s32HvBattCooltTReq]
  sTmSigProces_D_u8HvBattCoolgReq/1 -> [sTmSigProces_D_u8HvBattCoolgReq]
  sTmSigProces_Te_s32EvapFanFilter/1 -> [sTmSigProces_Te_s32EvapFanFilter]
  sTmSigProces_Te_s32HvBattCooltTFilter/1 -> [sTmSigProces_Te_s32HvBattCooltTFilter]
  [xTmComprCtrl_B_ModeChanged] -> SM3HPErr/5(xTmComprCtrl_B_ModeChanged)
  xTmComprCtrl_B_ModeChanged/1 -> [xTmComprCtrl_B_ModeChanged]

== system ScriptDemo/Create/createMerge/After/SM3SM23/SM3SM1Error ==
  sTmIn_Te_s32HvBattCooltTReq : Inport
  sTmSigProces_Te_s32HvBattCooltTFilter : Inport  Port=2
  "NegAndPosCheck " : Subsystem  AncestorBlock=CustomLib/TempNegAndPosCheck
  Terminator : Terminator
  rTmComprCtrl_Te_s32TempError : Outport  OutDataTypeStr=single
  wires:
  sTmSigProces_Te_s32HvBattCooltTFilter/1 -> "NegAndPosCheck "/2(Acture)
  "NegAndPosCheck "/2(Dvt_PosFlag) -> Terminator/1
  sTmIn_Te_s32HvBattCooltTReq/1 -> "NegAndPosCheck "/1(SetPoint)
  "NegAndPosCheck "/1(Dvt) -> rTmComprCtrl_Te_s32TempError/1

== system ScriptDemo/Create/createMerge/After/SM3SM23/SM3SM2Error ==
  note: 控制对象为低压饱和温度
  note: 控制对象为蒸发器温度滤波值
  sTmSigProces_Te_s32EvapFanReqRamp : Inport  OutDataTypeStr=single
  sTmDiag_D_u8TeEvapFltSt : Inport  Port=2  OutDataTypeStr=uint8
  sTmSigProces_Te_s32EvapFanFilter : Inport  Port=3  OutDataTypeStr=single
  sTmSigProces_Te_s32SatLp : Inport  Port=4  OutDataTypeStr=single
  yTmRefriModeMgr_B_CoolOCRMode : Inport  Port=5  OutDataTypeStr=boolean
  Add : Sum  Inputs=+-  OutDataTypeStr=single
  Compare To Constant : simulink/Logic and Bit Operations/Compare To Constant  relop===  const=1  OutDataTypeStr=boolean
  Constant : Constant  Value=3  OutDataTypeStr=single
  Constant2 : Constant  Value=cTmComprCtrl_Te_i16SatLpReplaceDiff  OutDataTypeStr=int16
  NegAndPosCheck 1 : Subsystem  AncestorBlock=CustomLib/TempNegAndPosCheck
  Saturation1 : Saturate  UpperLimit=12  LowerLimit=3
  Switch1 : Switch  Criteria=u2 ~= 0  SaturateOnIntegerOverflow=off  InputSameDT=off
  Switch2 : Switch  Criteria=u2 ~= 0  SaturateOnIntegerOverflow=off  InputSameDT=off
  Terminator : Terminator
  rTmComprCtrl_Te_s32TempError : Outport
  wires:
  [sTmDiag_D_u8TeEvapFltSt] -> Switch1/2
  [sTmSigProces_Te_s32SatLp] -> Add/1
  Constant2/1 -> Add/2
  Switch2/1 -> Saturation1/1
  NegAndPosCheck 1/2(Dvt_PosFlag) -> Terminator/1
  NegAndPosCheck 1/1(Dvt) -> rTmComprCtrl_Te_s32TempError/1
  Add/1 -> Switch1/1
  Saturation1/1 -> NegAndPosCheck 1/1(SetPoint)
  sTmSigProces_Te_s32EvapFanReqRamp/1 -> [sTmSigProces_Te_s32EvapFanReqRamp]  "sTmSigProces_Te_s32EvapFanReqRamp"
  sTmDiag_D_u8TeEvapFltSt/1 -> [sTmDiag_D_u8TeEvapFltSt]  "sTmDiag_D_u8TeEvapFltSt"
  sTmSigProces_Te_s32EvapFanFilter/1 -> [sTmSigProces_Te_s32EvapFanFilter]  "sTmSigProces_Te_s32EvapFanFilter"
  sTmSigProces_Te_s32SatLp/1 -> [sTmSigProces_Te_s32SatLp]  "sTmSigProces_Te_s32SatLp"
  [yTmRefriModeMgr_B_CoolOCRMode] -> Compare To Constant/1
  Compare To Constant/1 -> Switch2/2
  Constant/1 -> Switch2/1
  yTmRefriModeMgr_B_CoolOCRMode/1 -> [yTmRefriModeMgr_B_CoolOCRMode]  "yTmRefriModeMgr_B_CoolOCRMode"
  [sTmSigProces_Te_s32EvapFanReqRamp] -> Switch2/3
  [sTmSigProces_Te_s32EvapFanFilter] -> Switch1/3
  Switch1/1 -> NegAndPosCheck 1/2(Acture)

== system ScriptDemo/Create/createMerge/After/SM3SM23/SM3_Ki ==
  note: 等级1或2
  note: 等级3
  SM1Error : Inport
  SM2Error : Inport  Port=2
  sTmIn_D_u8DCChrgSt : Inport  Port=3  OutDataTypeStr=uint8
  sTmIn_D_u8HeatPump : Inport  Port=4  OutDataTypeStr=uint8
  sTmSigProces_Te_s32TAmb : Inport  Port=5  OutDataTypeStr=single
  sTmIn_X_s32ClimtRcirc : Inport  Port=6  OutDataTypeStr=single
  sTmComprCtrl_D_u8HvacFlowLevel : Inport  Port=7  OutDataTypeStr=uint8
  sTmSigProces_D_u8BattThermReq : Inport  Port=8  OutDataTypeStr=uint8
  sTmSigProces_D_u8HvBattCoolgReq : Inport  Port=9  OutDataTypeStr=uint8
  Add : Sum
  Add1 : Sum
  Compare To Constant : simulink/Logic and Bit Operations/Compare To Constant  relop===  const=3  OutDataTypeStr=boolean
  SM1Ki : Subsystem
  SM2Ki : Subsystem
  SM3SM1LikeKi : Subsystem
  SM3SM2LikeKi : Subsystem
  Switch : Switch  Criteria=u2 ~= 0  SaturateOnIntegerOverflow=off  InputSameDT=off
  Terminator : Terminator
  SM3Ki : Outport
  wires:
  [sTmIn_D_u8DCChrgSt] -> SM1Ki/2(sTmIn_D_u8DCChrgSt)
  [SM1Error] -> SM1Ki/4(Error)
  [sTmSigProces_D_u8HvBattCoolgReq] -> SM1Ki/3(sTmSigProces_D_u8HvBattCoolgReq)
  SM1Ki/1(SM1Ki) -> [SM1Ki]  "rTmComprCtrl_n_u16ComprRpmKiSM3SM1"
  [sTmSigProces_D_u8BattThermReq] -> SM1Ki/1(sTmSigProces_D_u8BattThermReq)
  [sTmComprCtrl_D_u8HvacFlowLevel] -> SM2Ki/4(sTmComprCtrl_D_u8HvacFlowLevel)
  [SM2Error] -> SM2Ki/1(Error)
  [sTmSigProces_Te_s32TAmb] -> SM2Ki/2(sTmSigProces_Te_s32TAmb)
  [sTmIn_X_s32ClimtRcirc] -> SM2Ki/3(sTmIn_X_s32ClimtRcirc)
  [sTmIn_X_s32ClimtRcirc] -> SM3SM2LikeKi/3(sTmIn_X_s32ClimtRcirc)
  SM3SM2LikeKi/1(Ki) -> [SM3SM2LikeKi]  "rTmComprCtrl_n_u16ComprRpmKiSM3SM2Like"
  [SM2Error] -> SM3SM2LikeKi/1(Error)
  [sTmSigProces_Te_s32TAmb] -> SM3SM2LikeKi/2(sTmSigProces_Te_s32TAmb)
  [sTmComprCtrl_D_u8HvacFlowLevel] -> SM3SM2LikeKi/4(sTmComprCtrl_D_u8HvacFlowLevel)
  SM3SM1LikeKi/1(Ki) -> [SM3SM1LikeKi]  "rTmComprCtrl_n_u16ComprRpmKiSM3SM1Like"
  [sTmSigProces_D_u8HvBattCoolgReq] -> SM3SM1LikeKi/3(sTmSigProces_D_u8HvBattCoolgReq)
  [sTmSigProces_D_u8BattThermReq] -> SM3SM1LikeKi/1(sTmSigProces_D_u8BattThermReq)
  [SM1Error] -> SM3SM1LikeKi/4(error)
  [sTmIn_D_u8DCChrgSt] -> SM3SM1LikeKi/2(sTmIn_D_u8DCChrgSt)
  SM1Error/1 -> [SM1Error]
  SM2Error/1 -> [SM2Error]
  sTmIn_D_u8DCChrgSt/1 -> [sTmIn_D_u8DCChrgSt]
  sTmIn_D_u8HeatPump/1 -> [sTmIn_D_u8HeatPump]
  sTmSigProces_Te_s32TAmb/1 -> [sTmSigProces_Te_s32TAmb]
  sTmIn_X_s32ClimtRcirc/1 -> [sTmIn_X_s32ClimtRcirc]
  sTmComprCtrl_D_u8HvacFlowLevel/1 -> [sTmComprCtrl_D_u8HvacFlowLevel]
  sTmSigProces_D_u8BattThermReq/1 -> [sTmSigProces_D_u8BattThermReq]
  sTmSigProces_D_u8HvBattCoolgReq/1 -> [sTmSigProces_D_u8HvBattCoolgReq]
  Add/1 -> Switch/3
  [SM3SM1LikeKi] -> Add/2
  [SM2Ki] -> Add/1
  [SM3SM2LikeKi] -> Add1/2
  [SM1Ki] -> Add1/1
  [sTmSigProces_D_u8HvBattCoolgReq] -> Compare To Constant/1
  Compare To Constant/1 -> Switch/2
  Switch/1 -> SM3Ki/1
  [sTmIn_D_u8HeatPump] -> Terminator/1
  Add1/1 -> Switch/1
  SM2Ki/1(SM2Ki) -> [SM2Ki]  "rTmComprCtrl_n_u16ComprRpmKiSM3SM2"

== system ScriptDemo/Create/createMerge/After/SM3SM23/SM3_Kp ==
  note: 等级1或2
  note: 等级3
  SM1Error : Inport
  SM2Error : Inport  Port=2
  sTmIn_D_u8DCChrgSt : Inport  Port=3  OutDataTypeStr=uint8
  sTmIn_D_u8HeatPump : Inport  Port=4  OutDataTypeStr=uint8
  sTmSigProces_Te_s32TAmb : Inport  Port=5  OutDataTypeStr=single
  sTmIn_X_s32ClimtRcirc : Inport  Port=6  OutDataTypeStr=single
  sTmComprCtrl_D_u8HvacFlowLevel : Inport  Port=7  OutDataTypeStr=uint8
  sTmSigProces_D_u8BattThermReq : Inport  Port=8  OutDataTypeStr=uint8
  sTmSigProces_D_u8HvBattCoolgReq : Inport  Port=9  OutDataTypeStr=uint8
  Add : Sum
  Add1 : Sum
  Compare To Constant : simulink/Logic and Bit Operations/Compare To Constant  relop===  const=3  OutDataTypeStr=boolean
  SM1Kp : Subsystem
  SM2Kp : Subsystem
  SM3SM1LikeKp : Subsystem
  SM3SM2LikeKp : Subsystem
  Switch : Switch  Criteria=u2 ~= 0  SaturateOnIntegerOverflow=off  InputSameDT=off
  Terminator : Terminator
  SM3Kp : Outport
  wires:
  [SM1Error] -> SM3SM1LikeKp/4(error)
  Switch/1 -> SM3Kp/1
  SM1Kp/1(SM1Kp) -> [SM1Kp]  "rTmComprCtrl_n_u16ComprRpmKpSM3SM1"
  [SM1Error] -> SM1Kp/4(Error)
  [sTmIn_D_u8DCChrgSt] -> SM1Kp/2(sTmIn_D_u8DCChrgSt)
  [sTmSigProces_D_u8HvBattCoolgReq] -> SM1Kp/3(sTmSigProces_D_u8HvBattCoolgReq)
  [sTmSigProces_D_u8BattThermReq] -> SM1Kp/1(sTmSigProces_D_u8BattThermReq)
  [SM2Error] -> SM2Kp/1(Error)
  [sTmComprCtrl_D_u8HvacFlowLevel] -> SM2Kp/4(sTmComprCtrl_D_u8HvacFlowLevel)
  [sTmIn_X_s32ClimtRcirc] -> SM2Kp/3(sTmIn_X_s32ClimtRcirc)
  [sTmSigProces_Te_s32TAmb] -> SM2Kp/2(sTmSigProces_Te_s32TAmb)
  SM3SM1LikeKp/1(Kp) -> [SM3SM1LikeKp]  "rTmComprCtrl_n_u16ComprRpmKpSM3SM1Like"
  [sTmSigProces_D_u8BattThermReq] -> SM3SM1LikeKp/1(sTmSigProces_D_u8BattThermReq)
  [sTmIn_D_u8DCChrgSt] -> SM3SM1LikeKp/2(sTmIn_D_u8DCChrgSt)
  [sTmSigProces_D_u8HvBattCoolgReq] -> SM3SM1LikeKp/3(sTmSigProces_D_u8HvBattCoolgReq)
  [SM2Kp] -> Add/1
  [SM3SM1LikeKp] -> Add/2
  SM1Error/1 -> [SM1Error]
  SM2Error/1 -> [SM2Error]
  sTmIn_D_u8DCChrgSt/1 -> [sTmIn_D_u8DCChrgSt]
  sTmIn_D_u8HeatPump/1 -> [sTmIn_D_u8HeatPump]
  sTmSigProces_Te_s32TAmb/1 -> [sTmSigProces_Te_s32TAmb]
  sTmIn_X_s32ClimtRcirc/1 -> [sTmIn_X_s32ClimtRcirc]
  sTmComprCtrl_D_u8HvacFlowLevel/1 -> [sTmComprCtrl_D_u8HvacFlowLevel]
  sTmSigProces_D_u8BattThermReq/1 -> [sTmSigProces_D_u8BattThermReq]
  sTmSigProces_D_u8HvBattCoolgReq/1 -> [sTmSigProces_D_u8HvBattCoolgReq]
  [sTmIn_X_s32ClimtRcirc] -> SM3SM2LikeKp/3(sTmIn_X_s32ClimtRcirc)
  [sTmComprCtrl_D_u8HvacFlowLevel] -> SM3SM2LikeKp/4(sTmComprCtrl_D_u8HvacFlowLevel)
  [SM2Error] -> SM3SM2LikeKp/1(Error)
  [sTmSigProces_Te_s32TAmb] -> SM3SM2LikeKp/2(sTmSigProces_Te_s32TAmb)
  SM3SM2LikeKp/1(Kp) -> [SM3SM2LikeKp]  "rTmComprCtrl_n_u16ComprRpmKpSM3SM2Like"
  [sTmSigProces_D_u8HvBattCoolgReq] -> Compare To Constant/1
  [sTmIn_D_u8HeatPump] -> Terminator/1
  Compare To Constant/1 -> Switch/2
  [SM3SM2LikeKp] -> Add1/2
  [SM1Kp] -> Add1/1
  Add1/1 -> Switch/1
  Add/1 -> Switch/3
  SM2Kp/1(SM2Kp) -> [SM2Kp]  "rTmComprCtrl_n_u16ComprRpmKpSM3SM2"

== system ScriptDemo/Create/createMerge/After/SM4/ID26259_SM4Error ==
  note: 制冷是实际-请求
      | 这里制热是请求-实际
  note: 未实现
      | 暖风芯体背风温度目标值∈[30, 60] ℃ 。
  note: 无PTC补热
  note: PTC 补热模式
  sTmSigProces_Te_s32SatHp : Inport
  yTmHvchCtrl_B_HpcPtcEnad : Inport  Port=2
  sTmSigProces_Te_s32HeatrAirTReqRamp : Inport  Port=3
  sTmSigProces_Te_s32HvacHexAirTFilter : Inport  Port=4
  Add2 : Sum
  Constant5 : Constant  Value=cTmComprCtrl_Te_i16HpReqTempSaturoffset
  NegAndPosCheck 4 : Subsystem  AncestorBlock=CustomLib/TempNegAndPosCheck
  NegAndPosCheck 5 : Subsystem  AncestorBlock=CustomLib/TempNegAndPosCheck
  Saturation3 : Saturate  UpperLimit=70  LowerLimit=15
  Switch2 : Switch  Criteria=u2 ~= 0  SaturateOnIntegerOverflow=off  InputSameDT=off
  Terminator : Terminator
  Terminator1 : Terminator
  Unary Minus : UnaryMinus
  rTmComprCtrl_Te_s32TempError : Outport
  wires:
  sTmSigProces_Te_s32SatHp/1 -> NegAndPosCheck 4/2(Acture)
  NegAndPosCheck 5/1(Dvt) -> Switch2/3
  sTmSigProces_Te_s32HeatrAirTReqRamp/1 -> Saturation3/1
  Switch2/1 -> Unary Minus/1
  NegAndPosCheck 5/2(Dvt_PosFlag) -> Terminator/1
  NegAndPosCheck 4/1(Dvt) -> Switch2/1
  Constant5/1 -> Add2/1
  NegAndPosCheck 4/2(Dvt_PosFlag) -> Terminator1/1
  sTmSigProces_Te_s32HvacHexAirTFilter/1 -> NegAndPosCheck 5/2(Acture)
  yTmHvchCtrl_B_HpcPtcEnad/1 -> Switch2/2
  Saturation3/1 -> Add2/2, NegAndPosCheck 5/1(SetPoint)
  Add2/1 -> NegAndPosCheck 4/1(SetPoint)
  Unary Minus/1 -> rTmComprCtrl_Te_s32TempError/1
